simulink model "part2"  (R2018b)
settings: Solver=VariableStepAuto  StartTime=0.0  StopTime=35  FixedStep=0.01  MaxStep=0.01  RelTol=1e-3
undefined symbols (not defined in the file or in its folder): D, DiscIntNeverNeededParam
libraries: simulink x8, Solver_SF x1, dsparch4 x1
(part 1 of 2)
settings Model: Creator=Hiro  LastModifiedBy=Lenovo
settings SolverCC: AlgebraicLoopSolver=LineSearch

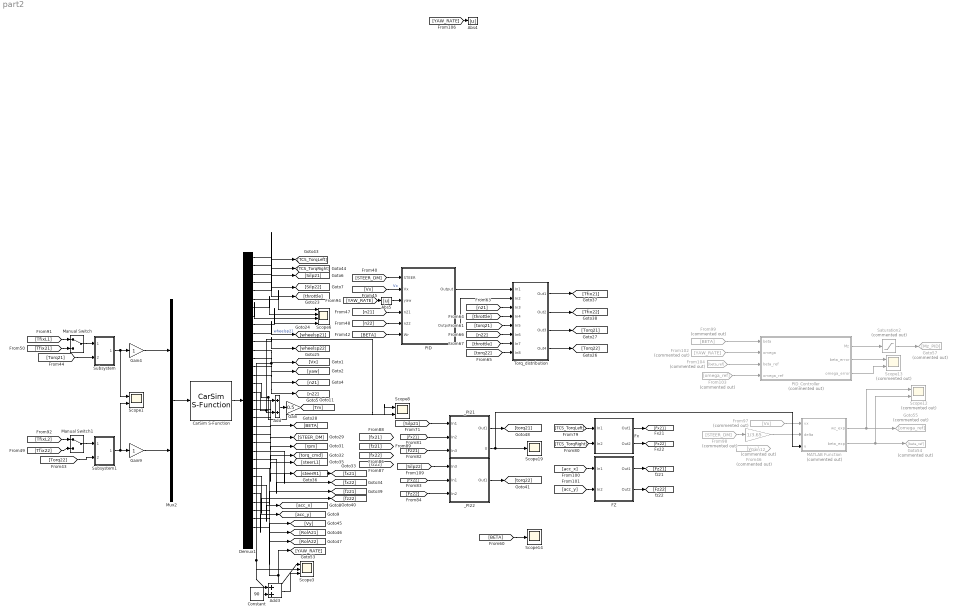
== system part2 ==
  Abs4 : Abs
  Abs5 : Abs
  Add : Sum
  Add3 : Sum
  CarSim S-Function : Solver_SF/CarSim S-Function  Priority=1  SIMFILE=simfile.sim  Run_RTs=off  vs_state_ind=Run  StopMode_ind=Vehicle Model
  Constant : Constant  Value=90
  Demux1 : Demux  Outputs=35
  FZ : Subsystem
  From102 : From  Commented=on  GotoTag=YAW_RATE
  From103 : From  Commented=on  GotoTag=omega_ref
  From104 : From  Commented=on  GotoTag=beta_ref
  From46 : From  Commented=on  GotoTag=yaw
  From97 : From  Commented=on  GotoTag=Vx
  From98 : From  Commented=on  GotoTag=STEER_DM
  From99 : From  Commented=on  GotoTag=BETA
  Fx : Subsystem
  Gain : Gain  Gain=0.5
  Gain12 : Gain  Commented=on  Gain=1/3.65
  Gain4 : Gain
  Gain9 : Gain
  Goto54 : Goto  Commented=on  GotoTag=beta_ref
  Goto55 : Goto  Commented=on  GotoTag=omega_ref
  Goto57 : Goto  Commented=on  GotoTag=Mz_PID
  MATLAB Function : MATLAB Function  Commented=on  TreatAsAtomicUnit=on
  Manual Switch : ManualSwitch
  Manual Switch1 : ManualSwitch
  Mux2 : Mux  Inputs=2
  PID : Subsystem
  PID_Controller : Subsystem  Commented=on
  Saturation2 : Saturate  Commented=on  UpperLimit=2000  LowerLimit=-2000
  Scope1 : Scope  NumInputPorts=2
  Scope12 : Scope  Commented=on  NumInputPorts=2
  Scope13 : Scope  Commented=on  NumInputPorts=2
  Scope14 : Scope
  Scope19 : Scope
  Scope3 : Scope  NumInputPorts=3
  Scope6 : Scope  NumInputPorts=4
  Scope8 : Scope  NumInputPorts=2
  Subsystem : Subsystem
  Subsystem1 : Subsystem
  Torq_distribution : Subsystem
  _PI21 : Subsystem
  _PI22 : Subsystem
  wires:
  CarSim S-Function/1 -> Demux1/1
  Demux1/4 -> [Silp22]
  Demux1/2 -> [TCS_TorqRight]
  Mux2/1 -> CarSim S-Function/1
  Demux1/5 -> [throttle]
  Demux1/6 -> Scope6/1
  Demux1/7 -> Scope6/2
  Demux1/8 -> Scope6/3
  Demux1/9 -> Scope6/4
  Demux1/10 -> [wheelsp21]  "wheelsp21"
  Demux1/11 -> [wheelsp22]
  Demux1/13 -> Add3/1, Scope3/2, [yaw]
  Demux1/14 -> [n21]
  Demux1/15 -> [n22]
  Demux1/17 -> Scope8/2, Add/2
  Demux1/16 -> Scope8/1, Add/1
  Gain/1 -> [Tm]
  Add/1 -> Gain/1
  [Vx] -> PID/2(Vx)  "Vx"
  [n21] -> PID/4(n21)
  [n22] -> PID/5(n22)
  Demux1/18 -> [BETA]
  Demux1/19 -> [STEER_DM]
  [STEER_DM] -> PID/1(STEER)
  Demux1/12 -> [Vx]
  Demux1/20 -> [rpm]
  Demux1/21 -> [torq_cmd]
  Demux1/22 -> [steerL1]
  Demux1/23 -> [steerR1]
  Demux1/24 -> [fx21]
  Demux1/25 -> [fx22]
  Demux1/26 -> [fz21]
  Demux1/27 -> [fz22]
  [n21] -> Torq_distribution/3(In3)
  [throttle] -> Torq_distribution/4(In4)
  [torq21] -> Torq_distribution/5(In5)
  [n22] -> Torq_distribution/6(In6)
  [throttle] -> Torq_distribution/7(In7)
  [torq22] -> Torq_distribution/8(In8)
  Demux1/1 -> [TCS_TorqLeft]
  Demux1/28 -> [acc_x]
  Demux1/29 -> [acc_y]
  Demux1/30 -> [Vy]
  [acc_x] -> FZ/1(In1)
  [acc_y] -> FZ/2(In2)
  FZ/2(Out2) -> [Fz22]
  Demux1/31 -> [RolA21]
  Demux1/32 -> [RolA22]
  [TCS_TorqLeft] -> Fx/1(In1)
  [TCS_TorqRight] -> Fx/2(In2)
  Fx/2(Out2) -> [Fx22]
  [Silp22] -> _PI22/1(In3)
  FZ/1(Out1) -> [Fz21]
  Torq_distribution/3(Out3) -> [Torq21]
  Torq_distribution/4(Out4) -> [Torq22]
  [Torq21] -> Subsystem/2(In2)
  Torq_distribution/1(Out1) -> [Tfix21]
  Torq_distribution/2(Out2) -> [Tfix22]
  PID/1(Output) -> Torq_distribution/1(In1)
  PID/2(Output1) -> Torq_distribution/2(In2)
  Subsystem/1(Out1) -> Scope1/1, Gain4/1
  Subsystem1/1(Out1) -> Scope1/2, Gain9/1
  Gain4/1 -> Mux2/1
  Gain9/1 -> Mux2/2
  Demux1/33 -> Scope3/1, [YAW_RATE]
  Constant/1 -> Add3/2
  Add3/1 -> Scope3/3
  [BETA] -> PID/6(Wr)
  Demux1/3 -> [Silp21]
  [Silp21] -> _PI21/1(In1)
  [Fx21] -> _PI21/2(In2)
  From97/1 -> MATLAB Function/1(vx)
  MATLAB Function/2(beta_exp) -> Scope12/2, Goto54/1
  MATLAB Function/1(wz_exp) -> Scope12/1, Goto55/1
  From98/1 -> Gain12/1
  PID_Controller/2(beta_error) -> Scope13/1
  PID_Controller/1(Mz) -> Saturation2/1
  PID_Controller/3(omega_error) -> Scope13/2
  Saturation2/1 -> Goto57/1
  From99/1 -> PID_Controller/1(beta)
  From102/1 -> PID_Controller/2(omega)
  From103/1 -> PID_Controller/4(omega_ref)
  From104/1 -> PID_Controller/3(beta_ref)
  Gain12/1 -> MATLAB Function/2(delta)
  [YAW_RATE] -> Abs4/1
  [YAW_RATE] -> Abs5/1
  [Tfix21] -> Manual Switch/2
  [Tfix22] -> Manual Switch1/2
  [Torq22] -> Subsystem1/2(In2)
  [TfixL2] -> Manual Switch1/1
  [TfixL1] -> Manual Switch/1
  Manual Switch/1 -> Subsystem/1(In1)
  Manual Switch1/1 -> Subsystem1/1(In1)
  _PI21/2(U) -> MATLAB Function/3(u), Scope19/1
  Fx/1(Out1) -> [Fx21]
  [Fz21] -> _PI21/3(In3)
  [Fx22] -> _PI22/2(In1)
  [Fz22] -> _PI22/3(In2)
  _PI21/1(Out1) -> [torq21]
  _PI22/1(Out1) -> [torq22]
  [BETA] -> Scope14/1
  Abs5/1 -> PID/3(yaw)

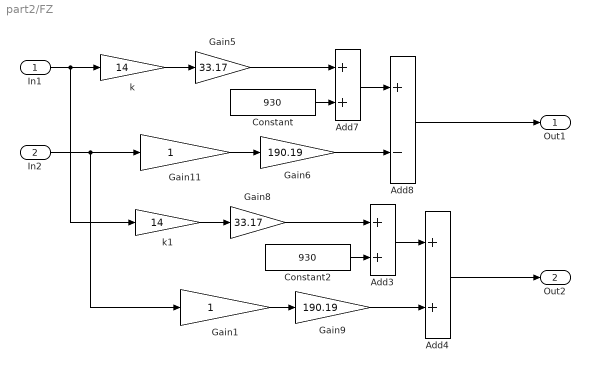
== system part2/FZ ==
  In1 : Inport
  In2 : Inport  Port=2
  Add3 : Sum
  Add4 : Sum
  Add7 : Sum
  Add8 : Sum  Inputs=+-
  Constant : Constant  Value=930
  Constant2 : Constant  Value=930
  Gain1 : Gain
  Gain11 : Gain
  Gain5 : Gain  Gain=33.17
  Gain6 : Gain  Gain=190.19
  Gain8 : Gain  Gain=33.17
  Gain9 : Gain  Gain=190.19
  k : Gain  Gain=14
  k1 : Gain  Gain=14
  Out1 : Outport
  Out2 : Outport  Port=2
  wires:
  Constant/1 -> Add7/2
  Add7/1 -> Add8/1
  k/1 -> Gain5/1
  Gain5/1 -> Add7/1
  Gain6/1 -> Add8/2
  Gain11/1 -> Gain6/1
  Add8/1 -> Out1/1
  In1/1 -> k1/1, k/1
  Gain1/1 -> Gain9/1
  Gain9/1 -> Add4/2
  Gain8/1 -> Add3/1
  k1/1 -> Gain8/1
  In2/1 -> Gain1/1, Gain11/1
  Add3/1 -> Add4/1
  Constant2/1 -> Add3/2
  Add4/1 -> Out2/1

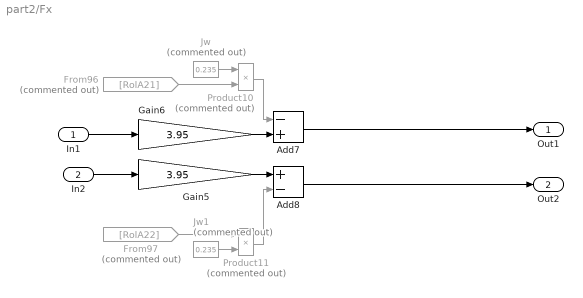
== system part2/Fx ==
  In1 : Inport
  In2 : Inport  Port=2
  Add7 : Sum  Inputs=-+
  Add8 : Sum  Inputs=+-
  From96 : From  Commented=on  GotoTag=RolA21
  From97 : From  Commented=on  GotoTag=RolA22
  Gain5 : Gain  Gain=3.95
  Gain6 : Gain  Gain=3.95
  Jw : Constant  Commented=on  Value=0.235
  Jw1 : Constant  Commented=on  Value=0.235
  Product10 : Product  Commented=on
  Product11 : Product  Commented=on
  Out1 : Outport
  Out2 : Outport  Port=2
  wires:
  From96/1 -> Product10/2
  Gain5/1 -> Add8/1
  Product11/1 -> Add8/2
  Gain6/1 -> Add7/2
  Jw/1 -> Product10/1
  Jw1/1 -> Product11/2
  Product10/1 -> Add7/1
  From97/1 -> Product11/1
  In2/1 -> Gain5/1
  In1/1 -> Gain6/1
  Add7/1 -> Out1/1
  Add8/1 -> Out2/1

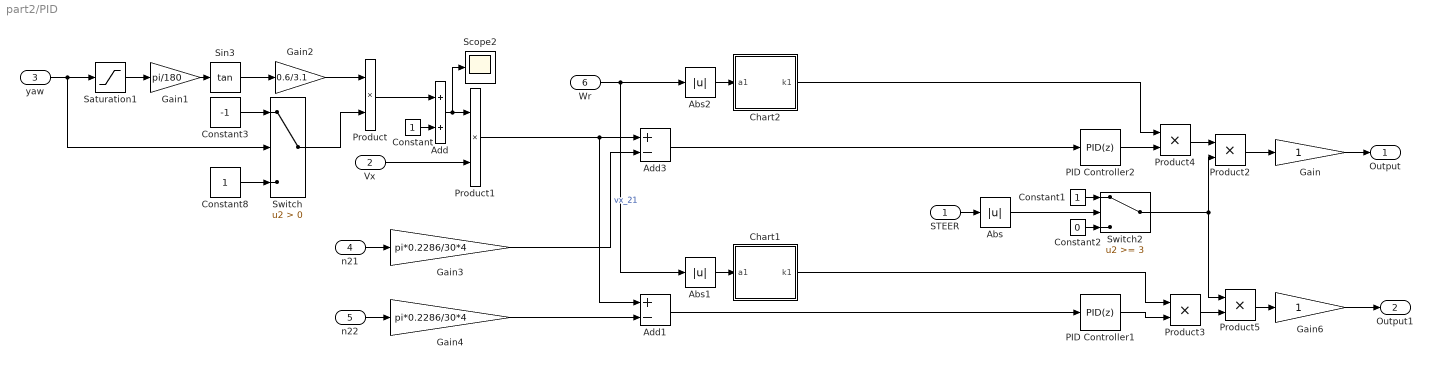
== system part2/PID ==
  STEER : Inport
  Vx : Inport  Port=2
  yaw : Inport  Port=3
  n21 : Inport  Port=4
  n22 : Inport  Port=5
  Wr : Inport  Port=6
  Abs : Abs
  Abs1 : Abs
  Abs2 : Abs
  Add : Sum
  Add1 : Sum  Inputs=+-
  Add3 : Sum  Inputs=+-
  Chart1 : Stateflow chart  TreatAsAtomicUnit=on
  Chart2 : Stateflow chart  TreatAsAtomicUnit=on
  Constant : Constant
  Constant1 : Constant
  Constant2 : Constant  Value=0
  Constant3 : Constant  Value=-1
  Constant8 : Constant
  Gain : Gain
  Gain1 : Gain  Gain=pi/180
  Gain2 : Gain  Gain=0.6/3.1
  Gain3 : Gain  Gain=pi*0.2286/30*4
  Gain4 : Gain  Gain=pi*0.2286/30*4
  Gain6 : Gain
  PID Controller1 : simulink/Continuous/PID Controller  Controller=PID  Form=Parallel  TimeDomain=Discrete-time  SampleTime=0.01  IntegratorMethod=Forward Euler  FilterMethod=Forward Euler  ControllerParametersSource=internal  P=300  I=0.75  D=0.5  UseFilter=on  N=100  TunerSelectOption=Transfer Function Based (PID Tuner App)  InitialConditionSource=internal  InitialConditionForIntegrator=0  InitialConditionForFilter=0  DifferentiatorICPrevScaledInput=0  ExternalReset=none  TrackingMode=off  Kt=1  LimitOutput=off  UpperSaturationLimit=inf  LowerSaturationLimit=-inf  LinearizeAsGain=on  AntiWindupMode=none  Kb=1  POutMin=[]  POutMax=[]  IOutMin=[]  IOutMax=[]  DOutMin=[]  DOutMax=[]  NOutMin=[]  NOutMax=[]  SumOutMin=[]  SumOutMax=[]  SaturationOutMin=[]  SaturationOutMax=[]  PParamMin=[]  PParamMax=[]  IParamMin=[]  IParamMax=[]  DParamMin=[]  DParamMax=[]  NParamMin=[]  NParamMax=[]  KbParamMin=[]  KbParamMax=[]  KtParamMin=[]  KtParamMax=[]  KbOutMin=[]  KbOutMax=[]  KtOutMin=[]  KtOutMax=[]  IntegratorOutMin=[]  IntegratorOutMax=[]  FilterOutMin=[]  FilterOutMax=[]  SumI1OutMin=[]  SumI1OutMax=[]  SumI2OutMin=[]  SumI2OutMax=[]  SumI3OutMin=[]  SumI3OutMax=[]  SumI4OutMin=[]  SumI4OutMax=[]  SumDOutMin=[]  SumDOutMax=[]  DifferentiatorOutMin=[]  DifferentiatorOutMax=[]  FilterDiffOutCoefMin=[]  FilterDiffOutCoefMax=[]  ReciprocalOutMin=[]  ReciprocalOutMax=[]  SumDenOutMin=[]  SumDenOutMax=[]  SumNumOutMin=[]  SumNumOutMax=[]  DivideOutMin=[]  DivideOutMax=[]  IntegratorContinuousStateAttributes=''  IntegratorStateMustResolveToSignalObject=off  IntegratorRTWStateStorageClass=Auto  FilterContinuousStateAttributes=''  FilterStateMustResolveToSignalObject=off  FilterRTWStateStorageClass=Auto  ParallelPVariant=InternalParameters  IdealPVariant=Disabled  IVariant=InternalParameters  DVariant=InternalParameters  IntegratorVariant=Discrete  SatVariant=Disabled  AWVariant=Passthrough  PCopyVariant=Disabled  TRVariant=Disabled  FdbkBlocksVariant=Forward  IdealPFdbkVariant=Disabled  SatFdbkVariant=Disabled  DerivativeFilterVariant=ForwardEulerFilter  NVariant=InternalParameters  NCopyVariant=Disabled  FilterICVariant=InternalICsFilter  IntegratorICVariant=InternalICs  ExternalResetVariant=Disabled  TRSumVariant=Passthrough  SumFdbkVariant=Disabled  SumVariant=Sum_PID
  PID Controller2 : simulink/Continuous/PID Controller  Controller=PID  Form=Parallel  TimeDomain=Discrete-time  SampleTime=0.01  IntegratorMethod=Forward Euler  FilterMethod=Forward Euler  ControllerParametersSource=internal  P=300  I=0.75  D=0.5  UseFilter=on  N=100  TunerSelectOption=Transfer Function Based (PID Tuner App)  InitialConditionSource=internal  InitialConditionForIntegrator=0  InitialConditionForFilter=0  DifferentiatorICPrevScaledInput=0  ExternalReset=none  TrackingMode=off  Kt=1  LimitOutput=off  UpperSaturationLimit=inf  LowerSaturationLimit=-inf  LinearizeAsGain=on  AntiWindupMode=none  Kb=1  POutMin=[]  POutMax=[]  IOutMin=[]  IOutMax=[]  DOutMin=[]  DOutMax=[]  NOutMin=[]  NOutMax=[]  SumOutMin=[]  SumOutMax=[]  SaturationOutMin=[]  SaturationOutMax=[]  PParamMin=[]  PParamMax=[]  IParamMin=[]  IParamMax=[]  DParamMin=[]  DParamMax=[]  NParamMin=[]  NParamMax=[]  KbParamMin=[]  KbParamMax=[]  KtParamMin=[]  KtParamMax=[]  KbOutMin=[]  KbOutMax=[]  KtOutMin=[]  KtOutMax=[]  IntegratorOutMin=[]  IntegratorOutMax=[]  FilterOutMin=[]  FilterOutMax=[]  SumI1OutMin=[]  SumI1OutMax=[]  SumI2OutMin=[]  SumI2OutMax=[]  SumI3OutMin=[]  SumI3OutMax=[]  SumI4OutMin=[]  SumI4OutMax=[]  SumDOutMin=[]  SumDOutMax=[]  DifferentiatorOutMin=[]  DifferentiatorOutMax=[]  FilterDiffOutCoefMin=[]  FilterDiffOutCoefMax=[]  ReciprocalOutMin=[]  ReciprocalOutMax=[]  SumDenOutMin=[]  SumDenOutMax=[]  SumNumOutMin=[]  SumNumOutMax=[]  DivideOutMin=[]  DivideOutMax=[]  IntegratorContinuousStateAttributes=''  IntegratorStateMustResolveToSignalObject=off  IntegratorRTWStateStorageClass=Auto  FilterContinuousStateAttributes=''  FilterStateMustResolveToSignalObject=off  FilterRTWStateStorageClass=Auto  ParallelPVariant=InternalParameters  IdealPVariant=Disabled  IVariant=InternalParameters  DVariant=InternalParameters  IntegratorVariant=Discrete  SatVariant=Disabled  AWVariant=Passthrough  PCopyVariant=Disabled  TRVariant=Disabled  FdbkBlocksVariant=Forward  IdealPFdbkVariant=Disabled  SatFdbkVariant=Disabled  DerivativeFilterVariant=ForwardEulerFilter  NVariant=InternalParameters  NCopyVariant=Disabled  FilterICVariant=InternalICsFilter  IntegratorICVariant=InternalICs  ExternalResetVariant=Disabled  TRSumVariant=Passthrough  SumFdbkVariant=Disabled  SumVariant=Sum_PID
  Product{,1..5} (6 alike) : Product
  Saturation1 : Saturate  UpperLimit=89.9  LowerLimit=-89.9
  Scope2 : Scope
  Sin3 : Trigonometry  Operator=tan
  Switch : Switch  Criteria=u2 > Threshold
  Switch2 : Switch  Threshold=3
  Output : Outport
  Output1 : Outport  Port=2
  wires:
  Constant3/1 -> Switch/1
  Constant8/1 -> Switch/3
  yaw/1 -> Switch/2, Saturation1/1
  Gain2/1 -> Product/1
  Switch/1 -> Product/2
  Product/1 -> Add/1
  Constant/1 -> Add/2
  Add/1 -> Scope2/1, Product1/1
  Vx/1 -> Product1/2
  n21/1 -> Gain3/1
  n22/1 -> Gain4/1
  Abs2/1 -> Chart2/1(a1)
  Abs1/1 -> Chart1/1(a1)
  Gain4/1 -> Add1/2
  Product1/1 -> Add1/1, Add3/1
  Gain3/1 -> Add3/2  "vx_21"
  Wr/1 -> Abs1/1, Abs2/1
  Gain/1 -> Output/1
  Gain6/1 -> Output1/1
  STEER/1 -> Abs/1
  PID Controller1/1 -> Product3/2
  PID Controller2/1 -> Product4/2
  Add3/1 -> PID Controller2/1
  Add1/1 -> PID Controller1/1
  Gain1/1 -> Sin3/1
  Sin3/1 -> Gain2/1
  Saturation1/1 -> Gain1/1
  Chart2/1(k1) -> Product4/1
  Chart1/1(k1) -> Product3/1
  Abs/1 -> Switch2/2
  Constant1/1 -> Switch2/1
  Switch2/1 -> Product2/2, Product5/1
  Constant2/1 -> Switch2/3
  Product2/1 -> Gain/1
  Product4/1 -> Product2/1
  Product5/1 -> Gain6/1
  Product3/1 -> Product5/2

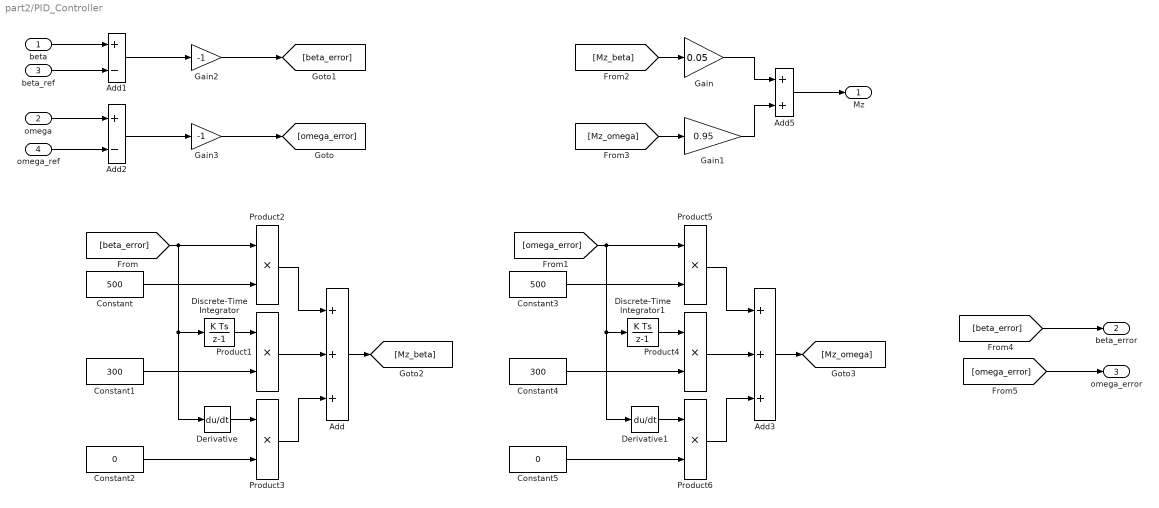
== system part2/PID_Controller ==
  beta : Inport
  omega : Inport  Port=2
  beta_ref : Inport  Port=3
  omega_ref : Inport  Port=4
  Add : Sum  Inputs=+++
  Add1 : Sum  Inputs=+-
  Add2 : Sum  Inputs=+-
  Add3 : Sum  Inputs=+++
  Add5 : Sum  Inputs=2
  Constant : Constant  Value=500
  Constant1 : Constant  Value=300
  Constant2 : Constant  Value=0
  Constant3 : Constant  Value=500
  Constant4 : Constant  Value=300
  Constant5 : Constant  Value=0
  Derivative : Derivative
  Derivative1 : Derivative
  Discrete-Time Integrator : DiscreteIntegrator  SampleTime=-1  ICPrevOutput=DiscIntNeverNeededParam  ICPrevScaledInput=DiscIntNeverNeededParam
  Discrete-Time Integrator1 : DiscreteIntegrator  SampleTime=-1  ICPrevOutput=DiscIntNeverNeededParam  ICPrevScaledInput=DiscIntNeverNeededParam
  Gain : Gain  Gain=0.05
  Gain1 : Gain  Gain=0.95
  Gain2 : Gain  Gain=-1
  Gain3 : Gain  Gain=-1
  Product{1..6} (6 alike) : Product
  Mz : Outport  VectorParamsAs1DForOutWhenUnconnected=on
  beta_error : Outport  Port=2  VectorParamsAs1DForOutWhenUnconnected=on
  omega_error : Outport  Port=3  VectorParamsAs1DForOutWhenUnconnected=on
  wires:
  Add2/1 -> Gain3/1
  beta/1 -> Add1/1
  omega_ref/1 -> Add2/2
  beta_ref/1 -> Add1/2
  omega/1 -> Add2/1
  Add1/1 -> Gain2/1
  [beta_error] -> Product2/1, Discrete-Time Integrator/1, Derivative/1
  Constant/1 -> Product2/2
  Product2/1 -> Add/1
  Constant1/1 -> Product1/2
  Discrete-Time Integrator/1 -> Product1/1
  Constant2/1 -> Product3/2
  Derivative/1 -> Product3/1
  Product1/1 -> Add/2
  Product3/1 -> Add/3
  Product5/1 -> Add3/1
  Discrete-Time Integrator1/1 -> Product4/1
  [omega_error] -> Product5/1, Discrete-Time Integrator1/1, Derivative1/1
  Constant5/1 -> Product6/2
  Product6/1 -> Add3/3
  Constant4/1 -> Product4/2
  Constant3/1 -> Product5/2
  Derivative1/1 -> Product6/1
  Product4/1 -> Add3/2
  Add/1 -> [Mz_beta]
  Add3/1 -> [Mz_omega]
  [Mz_beta] -> Gain/1
  Add5/1 -> Mz/1
  Gain/1 -> Add5/1
  [Mz_omega] -> Gain1/1
  Gain1/1 -> Add5/2
  Gain2/1 -> [beta_error]
  Gain3/1 -> [omega_error]
  [beta_error] -> beta_error/1
  [omega_error] -> omega_error/1

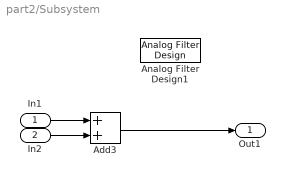
== system part2/Subsystem ==
  In1 : Inport
  In2 : Inport  Port=2
  Add3 : Sum
  Analog Filter Design1 : dsparch4/Analog Filter Design  method=Butterworth  filttype=Lowpass  N=6  Wlo=50  Whi=80  Rp=2  Rs=40
  Out1 : Outport
  wires:
  Add3/1 -> Out1/1
  In2/1 -> Add3/2
  In1/1 -> Add3/1

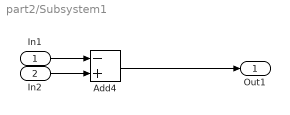
== system part2/Subsystem1 ==
  In1 : Inport
  In2 : Inport  Port=2
  Add4 : Sum  Inputs=-+
  Out1 : Outport
  wires:
  In2/1 -> Add4/2
  Add4/1 -> Out1/1
  In1/1 -> Add4/1

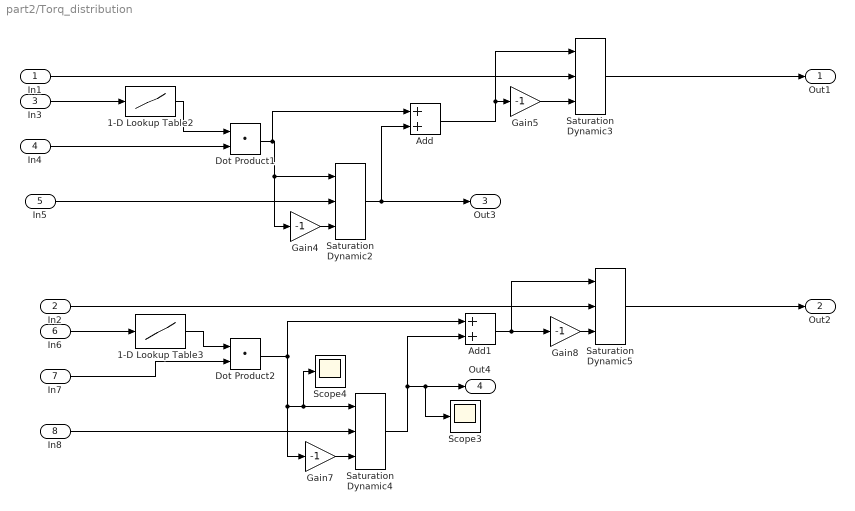
== system part2/Torq_distribution ==
  In1 : Inport
  In2 : Inport  Port=2
  In3 : Inport  Port=3
  In4 : Inport  Port=4
  In5 : Inport  Port=5
  In6 : Inport  Port=6
  In7 : Inport  Port=7
  In8 : Inport  Port=8
  1-D Lookup Table2 : Lookup_n-D  NumberOfTableDimensions=1  BreakpointsForDimension1=|  Table=|  InternalRulePriority=Speed  RndMeth=Simplest  InputSameDT=on
      BreakpointsForDimension1=|
      | [0
      | 256
      | 512
      | 768
      | 1024
      | 1280
      | 1536
      | 1792
      | 2048
      | 2304
      | 2560
      | 2816
      | 3072
      | 3328
      | 3584
      | 3840
      | 4096
      | 4352
      | 4608
      | 4864
      | 5120
      | 5376
      | 5632
      | ]
      Table=|
      | [140
      | 140
      | 140
      | 140
      | 140
      | 140
      | 140
      | 140
      | 140
      | 140
      | 140
      | 127
      | 116.75
      | 107.8
      | 99.952
      | 93.1085
      | 87.035
      | 81.973
      | 77.453
      | 73.4785
      | 69.935
      | 66.71
      | 63.685
      | ]
  1-D Lookup Table3 : Lookup_n-D  NumberOfTableDimensions=1  BreakpointsForDimension1=|  Table=|  InternalRulePriority=Speed  RndMeth=Simplest  InputSameDT=on
      BreakpointsForDimension1=|
      | [0
      | 256
      | 512
      | 768
      | 1024
      | 1280
      | 1536
      | 1792
      | 2048
      | 2304
      | 2560
      | 2816
      | 3072
      | 3328
      | 3584
      | 3840
      | 4096
      | 4352
      | 4608
      | 4864
      | 5120
      | 5376
      | 5632
      | ]
      Table=|
      | [140
      | 140
      | 140
      | 140
      | 140
      | 140
      | 140
      | 140
      | 140
      | 140
      | 140
      | 127
      | 116.75
      | 107.8
      | 99.952
      | 93.1085
      | 87.035
      | 81.973
      | 77.453
      | 73.4785
      | 69.935
      | 66.71
      | 63.685
      | ]
  Add : Sum
  Add1 : Sum
  Dot Product1 : DotProduct  InputSameDT=on  OutDataTypeStr=Inherit: Inherit via internal rule
  Dot Product2 : DotProduct  InputSameDT=on  OutDataTypeStr=Inherit: Inherit via internal rule
  Gain{4..5,7..8} (4 alike) : Gain  Gain=-1
  Saturation Dynamic{2..5} (4 alike) : simulink/Discontinuities/Saturation Dynamic  OutMin=[]  OutMax=[]  OutDataTypeStr=Inherit: Same as second input  OutDataType=fixdt(1, 16)  OutScaling=2^-10  DoSatur=off
  Scope3 : Scope
  Scope4 : Scope
  Out1 : Outport
  Out2 : Outport  Port=2
  Out3 : Outport  Port=3
  Out4 : Outport  Port=4
  wires:
  Saturation Dynamic5/1 -> Out2/1
  In4/1 -> Dot Product1/2
  1-D Lookup Table2/1 -> Dot Product1/1
  Saturation Dynamic2/1 -> Add/2, Out3/1
  Saturation Dynamic3/1 -> Out1/1
  In1/1 -> Saturation Dynamic3/2
  Gain5/1 -> Saturation Dynamic3/3
  Gain7/1 -> Saturation Dynamic4/3
  Gain8/1 -> Saturation Dynamic5/3
  Gain4/1 -> Saturation Dynamic2/3
  In2/1 -> Saturation Dynamic5/2
  In6/1 -> 1-D Lookup Table3/1
  In5/1 -> Saturation Dynamic2/2
  In3/1 -> 1-D Lookup Table2/1
  In7/1 -> Dot Product2/2
  In8/1 -> Saturation Dynamic4/2
  Dot Product1/1 -> Add/1, Gain4/1, Saturation Dynamic2/1
  Add/1 -> Saturation Dynamic3/1, Gain5/1
  Dot Product2/1 -> Gain7/1, Scope4/1, Saturation Dynamic4/1, Add1/1
  Add1/1 -> Saturation Dynamic5/1, Gain8/1
  Saturation Dynamic4/1 -> Add1/2, Scope3/1, Out4/1
  1-D Lookup Table3/1 -> Dot Product2/1

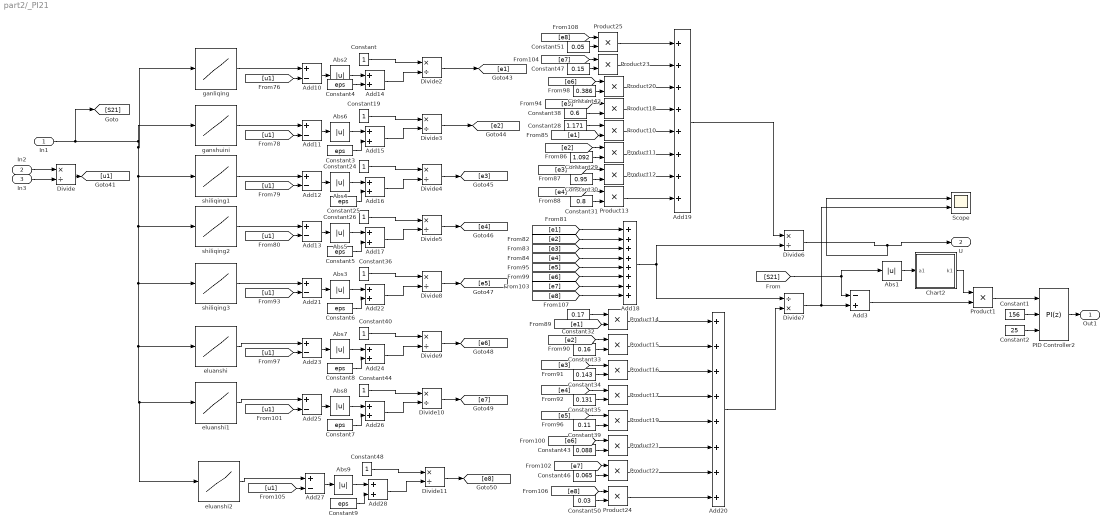
== system part2/_PI21 ==
  In1 : Inport
  In2 : Inport  Port=2
  In3 : Inport  Port=3
  Abs{1..9} (9 alike) : Abs
  Add{10..13,21,23,25,27} (8 alike) : Sum  Inputs=+-
  Add{14..17,22,24,26,28} (8 alike) : Sum
  Add18 : Sum  Inputs=++++++++
  Add19 : Sum  Inputs=++++++++
  Add20 : Sum  Inputs=++++++++
  Add3 : Sum  Inputs=-+
  Chart2 : Stateflow chart  TreatAsAtomicUnit=on
  Constant{,19,24,26,36,40,44,48} (8 alike) : Constant
  Constant1 : Constant  Value=156
  Constant2 : Constant  Value=25
  Constant{3..9,25} (8 alike) : Constant  Value=eps
  Constant28 : Constant  Value=1.171
  Constant29 : Constant  Value=1.092
  Constant30 : Constant  Value=0.95
  Constant31 : Constant  Value=0.8
  Constant32 : Constant  Value=0.17
  Constant33 : Constant  Value=0.16
  Constant34 : Constant  Value=0.143
  Constant35 : Constant  Value=0.131
  Constant38 : Constant  Value=0.6
  Constant39 : Constant  Value=0.11
  Constant42 : Constant  Value=0.386
  Constant43 : Constant  Value=0.088
  Constant46 : Constant  Value=0.065
  Constant47 : Constant  Value=0.15
  Constant50 : Constant  Value=0.03
  Constant51 : Constant  Value=0.05
  Divide{,2..6,8..11} (10 alike) : Product  Inputs=*/
  Divide7 : Product  Inputs=/*
  PID Controller2 : simulink/Continuous/PID Controller  Controller=PI  Form=Parallel  TimeDomain=Discrete-time  SampleTime=0.01  IntegratorMethod=Forward Euler  FilterMethod=Forward Euler  ControllerParametersSource=external  P=156  I=25  D=D  UseFilter=on  N=100  TunerSelectOption=Transfer Function Based (PID Tuner App)  InitialConditionSource=internal  InitialConditionForIntegrator=0  InitialConditionForFilter=0  DifferentiatorICPrevScaledInput=0  ExternalReset=none  TrackingMode=off  Kt=1  LimitOutput=on  UpperSaturationLimit=inf  LowerSaturationLimit=-inf  LinearizeAsGain=on  AntiWindupMode=clamping  Kb=1  POutMin=[]  POutMax=[]  IOutMin=[]  IOutMax=[]  DOutMin=[]  DOutMax=[]  NOutMin=[]  NOutMax=[]  SumOutMin=[]  SumOutMax=[]  SaturationOutMin=[]  SaturationOutMax=[]  PParamMin=[]  PParamMax=[]  IParamMin=[]  IParamMax=[]  DParamMin=[]  DParamMax=[]  NParamMin=[]  NParamMax=[]  KbParamMin=[]  KbParamMax=[]  KtParamMin=[]  KtParamMax=[]  KbOutMin=[]  KbOutMax=[]  KtOutMin=[]  KtOutMax=[]  IntegratorOutMin=[]  IntegratorOutMax=[]  FilterOutMin=[]  FilterOutMax=[]  SumI1OutMin=[]  SumI1OutMax=[]  SumI2OutMin=[]  SumI2OutMax=[]  SumI3OutMin=[]  SumI3OutMax=[]  SumI4OutMin=[]  SumI4OutMax=[]  SumDOutMin=[]  SumDOutMax=[]  DifferentiatorOutMin=[]  DifferentiatorOutMax=[]  FilterDiffOutCoefMin=[]  FilterDiffOutCoefMax=[]  ReciprocalOutMin=[]  ReciprocalOutMax=[]  SumDenOutMin=[]  SumDenOutMax=[]  SumNumOutMin=[]  SumNumOutMax=[]  DivideOutMin=[]  DivideOutMax=[]  IntegratorContinuousStateAttributes=''  IntegratorStateMustResolveToSignalObject=off  IntegratorRTWStateStorageClass=Auto  FilterContinuousStateAttributes=''  FilterStateMustResolveToSignalObject=off  FilterRTWStateStorageClass=Auto  ParallelPVariant=ExternalParameters  IdealPVariant=Disabled  IVariant=ExternalParameters  DVariant=Disabled  IntegratorVariant=Discrete  SatVariant=Enabled  AWVariant=DiscClampingParallel  PCopyVariant=Disabled  TRVariant=Disabled  FdbkBlocksVariant=Forward  IdealPFdbkVariant=Disabled  SatFdbkVariant=Disabled  DerivativeFilterVariant=Disabled  NVariant=Disabled  NCopyVariant=Disabled_SignalSpec  FilterICVariant=Disabled  IntegratorICVariant=InternalICs  ExternalResetVariant=Disabled  TRSumVariant=Passthrough  SumFdbkVariant=Disabled  SumVariant=Sum_PI
  Product{1,10..25} (17 alike) : Product
  Scope : Scope  NumInputPorts=2
  eluanshi : Lookup_n-D  NumberOfTableDimensions=1  BreakpointsForDimension1=[0.00591,0.009,0.01212,0.01856,0.0196,0.02707,0.03557,0.04385,0.05236,0.06524,0.1011,0.13927,0.18595,0.21975,0.26849,0.32574,0.38507,0.44646,0.51635,0.58188,0.63914,0.70697,0.78123,0.86792,0.92103,0.97184,0.993]  Table=[0.04929,0.12757,0.19671,0.25086,0.2838,0.31087,0.34088,0.36501,0.38001,0.38915,0.38915,0.38621,0.38295,0.37414,0.37121,0.36208,0.35588,0.34707,0.33794,0.335,0.32587,0.31707,0.31087,0.2988,0.29293,0.28673,0.2838]  InternalRulePriority=Speed  RndMeth=Simplest  InputSameDT=on
  eluanshi1 : Lookup_n-D  NumberOfTableDimensions=1  BreakpointsForDimension1=|  Table=|  InternalRulePriority=Speed  RndMeth=Simplest  InputSameDT=on
      BreakpointsForDimension1=|
      | [0.00154
      | 0.00798
      | 0.01649
      | 0.0227
      | 0.03121
      | 0.04178
      | 0.05673
      | 0.12433
      | 0.19216
      | 0.26642
      | 0.36598
      | 0.4952
      | 0.61591
      | 0.79388
      | 0.91873
      | 1.00357]
      Table=|
      | [0.04636
      | 0.11257
      | 0.14257
      | 0.17551
      | 0.18465
      | 0.19052
      | 0.19052
      | 0.18758
      | 0.18465
      | 0.17551
      | 0.17258
      | 0.16051
      | 0.15758
      | 0.14551
      | 0.13638
      | 0.1305]
  eluanshi2 : Lookup_n-D  NumberOfTableDimensions=1  BreakpointsForDimension1=|  Table=|  InternalRulePriority=Speed  RndMeth=Simplest  InputSameDT=on
      BreakpointsForDimension1=|
      | [0.00361
      | 0.00798
      | 0.01212
      | 0.01419
      | 0.01856
      | 0.0227
      | 0.02707
      | 0.02914
      | 0.04178
      | 0.09903
      | 0.15836
      | 0.26435
      | 0.37012
      | 0.49934
      | 0.60327
      | 0.69225
      | 0.78537
      | 0.86792
      | 0.94425
      | 1.0015]
      Table=|
      | [0.05549
      | 0.1093
      | 0.13964
      | 0.1517
      | 0.16051
      | 0.16964
      | 0.17845
      | 0.18465
      | 0.19052
      | 0.19052
      | 0.18465
      | 0.17845
      | 0.17258
      | 0.16671
      | 0.15758
      | 0.15464
      | 0.14551
      | 0.14257
      | 0.13638
      | 0.13344]
  ganliqing : Lookup_n-D  NumberOfTableDimensions=1  BreakpointsForDimension1=|  Table=|  InternalRulePriority=Speed  RndMeth=Simplest  InputSameDT=on
      BreakpointsForDimension1=|
      | [0.01498
      | 0.03128
      | 0.05446
      | 0.06846
      | 0.08017
      | 0.09165
      | 0.10335
      | 0.11506
      | 0.12424
      | 0.13595
      | 0.15454
      | 0.16625
      | 0.17772
      | 0.19632
      | 0.22202
      | 0.25691
      | 0.31499
      | 0.38017
      | 0.49196
      | 0.59433
      | 0.70129
      | 0.80367
      | 0.86885
      | 0.95493
      | 0.999]
      Table=|
      | [0.38854
      | 0.66554
      | 0.92268
      | 1.00503
      | 1.04474
      | 1.08738
      | 1.12058
      | 1.13686
      | 1.1502
      | 1.16322
      | 1.1668
      | 1.1668
      | 1.1668
      | 1.16322
      | 1.15346
      | 1.14044
      | 1.11049
      | 1.07762
      | 1.02489
      | 0.9689
      | 0.91617
      | 0.86019
      | 0.82699
      | 0.78435
      | 0.76123]
  ganshuini : Lookup_n-D  NumberOfTableDimensions=1  BreakpointsForDimension1=|  Table=|  InternalRulePriority=Speed  RndMeth=Simplest  InputSameDT=on
      BreakpointsForDimension1=|
      | [0
      | 0.00612
      | 0.01323
      | 0.0185
      | 0.024
      | 0.03293
      | 0.04531
      | 0.05241
      | 0.06295
      | 0.06845
      | 0.07555
      | 0.08266
      | 0.08976
      | 0.0932
      | 0.10213
      | 0.11107
      | 0.12161
      | 0.13055
      | 0.14315
      | 0.15369
      | 0.17156
      | 0.18577
      | 0.19631
      | 0.21419
      | 0.2355
      | 0.25497
      | 0.27468
      | 0.28889
      | 0.30676
      | 0.3173
      | 0.33334
      | 0.35465
      | 0.37252
      | 0.3991
      | 0.41858
      | 0.44539
      | 0.46143
      | 0.48985
      | 0.51299
      | 0.53613
      | 0.55194
      | 0.56798
      | 0.59823
      | 0.6161
      | 0.64085
      | 0.66926
      | 0.69424
      | 0.69791
      | 0.71211
      | 0.75107
      | 0.79209
      | 0.81706
      | 0.85075
      | 0.89887
      | 0.93599
      | 0.98411
      | 0.99832]
      Table=|
      | [0.0357
      | 0.13134
      | 0.30251
      | 0.41079
      | 0.52393
      | 0.63999
      | 0.78847
      | 0.84617
      | 0.90679
      | 0.9444
      | 0.97228
      | 0.99238
      | 1.01248
      | 1.02512
      | 1.04263
      | 1.05787
      | 1.06532
      | 1.07537
      | 1.07797
      | 1.08056
      | 1.08056
      | 1.07797
      | 1.07537
      | 1.06792
      | 1.05527
      | 1.05009
      | 1.04004
      | 1.03258
      | 1.02512
      | 1.01994
      | 1.00989
      | 0.99724
      | 0.98979
      | 0.97455
      | 0.9645
      | 0.94959
      | 0.94181
      | 0.92949
      | 0.91425
      | 0.90161
      | 0.89156
      | 0.8841
      | 0.86886
      | 0.86141
      | 0.84876
      | 0.82867
      | 0.81602
      | 0.81343
      | 0.80857
      | 0.78587
      | 0.76318
      | 0.75313
      | 0.73562
      | 0.70547
      | 0.69024
      | 0.66268
      | 0.6549]
  shiliqing1 : Lookup_n-D  NumberOfTableDimensions=1  BreakpointsForDimension1=|  Table=|  InternalRulePriority=Speed  RndMeth=Simplest  InputSameDT=on
      BreakpointsForDimension1=|
      | [0.00269
      | 0.00429
      | 0.01139
      | 0.01689
      | 0.02033
      | 0.0256
      | 0.0311
      | 0.04004
      | 0.04874
      | 0.06135
      | 0.07372
      | 0.08609
      | 0.0987
      | 0.11451
      | 0.13948
      | 0.1734
      | 0.20342
      | 0.23023
      | 0.24787
      | 0.26391
      | 0.28522
      | 0.30676
      | 0.3173
      | 0.35465
      | 0.39383
      | 0.42935
      | 0.47564
      | 0.51826
      | 0.55905
      | 0.59113
      | 0.63925
      | 0.68003
      | 0.72266
      | 0.7529
      | 0.79552
      | 0.84548
      | 0.89153
      | 0.92545
      | 0.99488]
      Table=|
      | [0.04835
      | 0.16927
      | 0.24707
      | 0.3278
      | 0.39328
      | 0.54662
      | 0.63221
      | 0.70547
      | 0.76059
      | 0.82607
      | 0.87405
      | 0.89901
      | 0.9243
      | 0.93694
      | 0.93954
      | 0.93694
      | 0.92689
      | 0.92171
      | 0.90906
      | 0.9042
      | 0.89415
      | 0.8841
      | 0.87665
      | 0.864
      | 0.84876
      | 0.82867
      | 0.81116
      | 0.79592
      | 0.77323
      | 0.75832
      | 0.74049
      | 0.72298
      | 0.70029
      | 0.69024
      | 0.67014
      | 0.64744
      | 0.62994
      | 0.6147
      | 0.58196]
  shiliqing2 : Lookup_n-D  NumberOfTableDimensions=1  BreakpointsForDimension1=|  Table=|  InternalRulePriority=Speed  RndMeth=Simplest  InputSameDT=on
      BreakpointsForDimension1=|
      | [8.52288E-4
      | 0.00429
      | 0.00612
      | 0.00796
      | 0.01139
      | 0.01506
      | 0.01689
      | 0.0185
      | 0.02033
      | 0.02216
      | 0.0256
      | 0.02927
      | 0.03454
      | 0.0382
      | 0.04164
      | 0.04714
      | 0.05058
      | 0.05768
      | 0.06478
      | 0.07189
      | 0.08082
      | 0.08793
      | 0.0932
      | 0.0987
      | 0.1058
      | 0.1129
      | 0.12528
      | 0.14315
      | 0.1876
      | 0.21052
      | 0.23023
      | 0.25337
      | 0.29072
      | 0.33678
      | 0.40437
      | 0.48435
      | 0.55561
      | 0.6035
      | 0.70662
      | 0.76894
      | 0.84364
      | 0.92018
      | 1.00015]
      Table=|
      | [0.04575
      | 0.09859
      | 0.14139
      | 0.19423
      | 0.24221
      | 0.285
      | 0.33525
      | 0.37059
      | 0.40074
      | 0.43348
      | 0.46622
      | 0.53171
      | 0.56672
      | 0.59201
      | 0.62475
      | 0.65231
      | 0.675
      | 0.71034
      | 0.73789
      | 0.75313
      | 0.77064
      | 0.77842
      | 0.78328
      | 0.78847
      | 0.79592
      | 0.79852
      | 0.79852
      | 0.79333
      | 0.78587
      | 0.77842
      | 0.77064
      | 0.76577
      | 0.75313
      | 0.73562
      | 0.71293
      | 0.68505
      | 0.66009
      | 0.64485
      | 0.6147
      | 0.58715
      | 0.56186
      | 0.53657
      | 0.50902]
  shiliqing3 : Lookup_n-D  NumberOfTableDimensions=1  BreakpointsForDimension1=|  Table=|  InternalRulePriority=Speed  RndMeth=Simplest  InputSameDT=on
      BreakpointsForDimension1=|
      | [0.0
      | 0.00154
      | 0.00798
      | 0.01212
      | 0.01419
      | 0.01856
      | 0.02477
      | 0.02914
      | 0.03764
      | 0.04615
      | 0.05236
      | 0.05673
      | 0.06087
      | 0.06937
      | 0.07788
      | 0.08846
      | 0.10317
      | 0.11812
      | 0.1372
      | 0.16893
      | 0.20503
      | 0.24941
      | 0.29171
      | 0.32988
      | 0.37012
      | 0.41243
      | 0.45496
      | 0.49083
      | 0.529
      | 0.57775
      | 0.62856
      | 0.68167
      | 0.73249
      | 0.77686
      | 0.82975
      | 0.90608
      | 0.94839
      | 1]
      Table=|
      | [0.0
      | 0.09756
      | 0.14551
      | 0.20878
      | 0.25379
      | 0.32
      | 0.35588
      | 0.39208
      | 0.44329
      | 0.47917
      | 0.50624
      | 0.5245
      | 0.5395
      | 0.55451
      | 0.57245
      | 0.58158
      | 0.59071
      | 0.59952
      | 0.59658
      | 0.59365
      | 0.58745
      | 0.57864
      | 0.57245
      | 0.56364
      | 0.55451
      | 0.54831
      | 0.5395
      | 0.53331
      | 0.5245
      | 0.51537
      | 0.5033
      | 0.49417
      | 0.48536
      | 0.47623
      | 0.46416
      | 0.44916
      | 0.44329
      | 0.43122]
  Out1 : Outport
  U : Outport  Port=2
  wires:
  [e3] -> Add18/3
  Divide2/1 -> [e1]
  Product17/1 -> Add20/4
  Divide/1 -> [u1]
  Add15/1 -> Divide3/2
  Constant19/1 -> Divide3/1
  Abs9/1 -> Add28/1
  [u1] -> Add13/2
  Add11/1 -> Abs6/1
  Add13/1 -> Abs5/1
  In1/1 -> [S21], eluanshi2/1, eluanshi1/1, eluanshi/1, shiliqing3/1, shiliqing2/1, shiliqing1/1, ganliqing/1, ganshuini/1
  Constant/1 -> Divide2/1
  ganliqing/1 -> Add10/1
  Constant46/1 -> Product22/2
  Constant24/1 -> Divide4/1
  Add12/1 -> Abs4/1
  Constant4/1 -> Add14/2
  [e3] -> Product12/1
  [e1] -> Product14/2
  [u1] -> Add21/2
  [u1] -> Add11/2
  Add16/1 -> Divide4/2
  Constant40/1 -> Divide9/1
  Abs4/1 -> Add16/1
  [e2] -> Add18/2
  [e2] -> Product11/1
  [e7] -> Product22/1
  Abs8/1 -> Add26/1
  Constant9/1 -> Add28/2
  Constant25/1 -> Add16/2
  Abs2/1 -> Add14/1
  Abs6/1 -> Add15/1
  Abs5/1 -> Add17/1
  [e4] -> Add18/4
  [e6] -> Product21/1
  Add17/1 -> Divide5/2
  Product18/1 -> Add19/4
  ganshuini/1 -> Add11/1
  Product12/1 -> Add19/7
  Constant31/1 -> Product13/2
  Product15/1 -> Add20/2
  shiliqing3/1 -> Add21/1
  Divide5/1 -> [e4]
  Constant26/1 -> Divide5/1
  [e5] -> Product18/1
  Divide9/1 -> [e6]
  Constant29/1 -> Product11/2
  Constant5/1 -> Add17/2
  Constant3/1 -> Add15/2
  Add14/1 -> Divide2/2
  Product13/1 -> Add19/8
  Constant42/1 -> Product20/2
  [e5] -> Add18/5
  Add23/1 -> Abs7/1
  Abs3/1 -> Add22/1
  Add19/1 -> Divide6/1
  Constant30/1 -> Product12/2
  Product10/1 -> Add19/5
  Constant34/1 -> Product16/2
  [u1] -> Add10/2
  [e6] -> Product20/1
  Divide3/1 -> [e2]
  [u1] -> Add12/2
  [e4] -> Product17/1
  Constant35/1 -> Product17/2
  Constant33/1 -> Product15/2
  [e2] -> Product15/1
  Constant38/1 -> Product18/2
  Constant44/1 -> Divide10/1
  eluanshi/1 -> Add23/1
  Constant6/1 -> Add22/2
  Add20/1 -> Divide7/2
  Constant8/1 -> Add24/2
  Abs7/1 -> Add24/1
  Constant39/1 -> Product19/2
  Constant7/1 -> Add26/2
  Product14/1 -> Add20/1
  Add22/1 -> Divide8/2
  Constant43/1 -> Product21/2
  Constant32/1 -> Product14/1
  [u1] -> Add23/2
  [e3] -> Product16/1
  [e4] -> Product13/1
  Add18/1 -> Divide7/1, Divide6/2
  Divide10/1 -> [e7]
  Add24/1 -> Divide9/2
  Constant47/1 -> Product23/2
  Add27/1 -> Abs9/1
  Constant51/1 -> Product25/2
  [u1] -> Add27/2
  [e1] -> Product10/2
  Constant36/1 -> Divide8/1
  Product16/1 -> Add20/3
  Add25/1 -> Abs8/1
  Product19/1 -> Add20/5
  Add28/1 -> Divide11/2
  Product11/1 -> Add19/6
  Add26/1 -> Divide10/2
  Add21/1 -> Abs3/1
  Divide4/1 -> [e3]
  [e7] -> Product23/1
  [e8] -> Product24/1
  Constant50/1 -> Product24/2
  [u1] -> Add25/2
  [e8] -> Product25/1
  Product21/1 -> Add20/6
  Add10/1 -> Abs2/1
  eluanshi1/1 -> Add25/1
  Constant48/1 -> Divide11/1
  Constant28/1 -> Product10/1
  shiliqing1/1 -> Add12/1
  Divide11/1 -> [e8]
  [e5] -> Product19/1
  Divide8/1 -> [e5]
  shiliqing2/1 -> Add13/1
  eluanshi2/1 -> Add27/1
  In3/1 -> Divide/2
  In2/1 -> Divide/1
  Add3/1 -> Product1/2
  Product1/1 -> PID Controller2/1
  Abs1/1 -> Chart2/1(a1)
  Chart2/1(k1) -> Product1/1
  Product20/1 -> Add19/3
  [e6] -> Add18/6
  [e1] -> Add18/1
  Constant1/1 -> PID Controller2/2
  Constant2/1 -> PID Controller2/3
  [S21] -> Add3/1, Abs1/1
  Divide7/1 -> Scope/2, Add3/2
  PID Controller2/1 -> Out1/1
  Divide6/1 -> U/1, Scope/1
  Product23/1 -> Add19/2
  Product22/1 -> Add20/7
  [e7] -> Add18/7
  Product24/1 -> Add20/8
  [e8] -> Add18/8
  Product25/1 -> Add19/1
